simulink model "Tisch"  (R2016b)
settings: Solver=VariableStepAuto  StartTime=0.0  StopTime=5  RelTol=1e-3
settings Model: Creator=fabienlapok  LastModifiedBy=fabienlapok

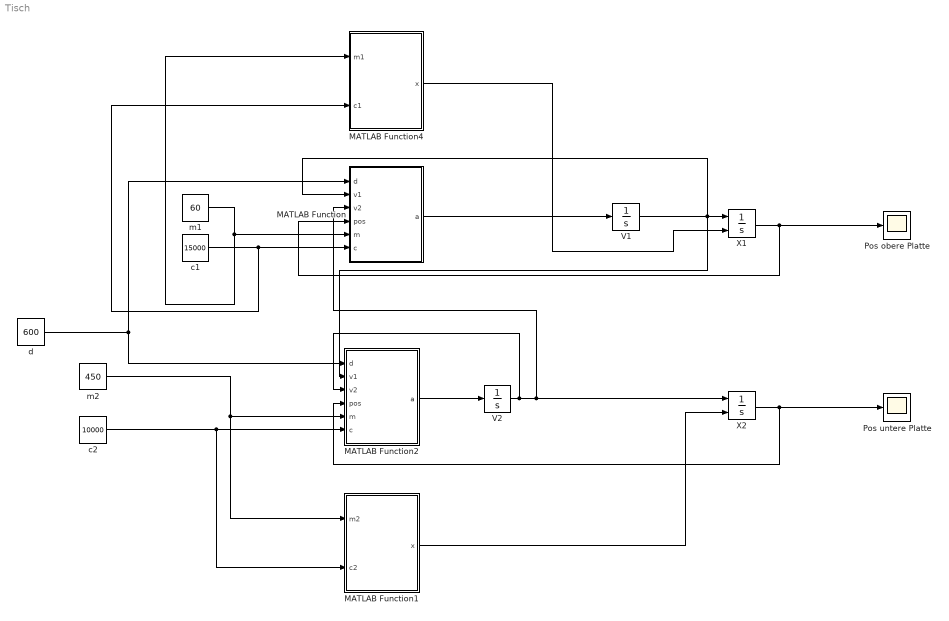
== system Tisch ==
  MATLAB Function : MATLAB Function  TreatAsAtomicUnit=on
  MATLAB Function1 : MATLAB Function  TreatAsAtomicUnit=on
  MATLAB Function2 : MATLAB Function  TreatAsAtomicUnit=on
  MATLAB Function4 : MATLAB Function  TreatAsAtomicUnit=on
  Pos obere Platte : Scope
  Pos untere Platte : Scope
  V1 : Integrator
  V2 : Integrator
  X1 : Integrator  InitialConditionSource=external
  X2 : Integrator  InitialConditionSource=external
  c1 : Constant  Value=15000
  c2 : Constant  Value=10000
  d : Constant  Value=600
  m1 : Constant  Value=60
  m2 : Constant  Value=450
  wires:
  MATLAB Function2/1(a) -> V2/1
  V2/1 -> MATLAB Function2/3(v2), MATLAB Function/3(v2), X2/1
  MATLAB Function/1(a) -> V1/1
  d/1 -> MATLAB Function/1(d), MATLAB Function2/1(d)
  m1/1 -> MATLAB Function4/1(m1), MATLAB Function/5(m)
  m2/1 -> MATLAB Function1/1(m2), MATLAB Function2/5(m)
  c1/1 -> MATLAB Function4/2(c1), MATLAB Function/6(c)
  c2/1 -> MATLAB Function1/2(c2), MATLAB Function2/6(c)
  X2/1 -> Pos untere Platte/1, MATLAB Function2/4(pos)
  X1/1 -> MATLAB Function/4(pos), Pos obere Platte/1
  MATLAB Function4/1(x) -> X1/2
  MATLAB Function1/1(x) -> X2/2
  V1/1 -> MATLAB Function2/2(v1), X1/1, MATLAB Function/2(v1)

== matlab function Tisch/MATLAB Function1 ==
  data: x output; m2 input; c2 input
function x = RuheposM2(m2, c2)
%Funktion zur Berechnung der Ruheposition der ersten (oberen) Platte 
    g= -9.81;
    
    x = m2*g/(2*c2); %[m]

== matlab function Tisch/MATLAB Function ==
  data: d input; a output; v1 input; v2 input; pos input; m input; c input
function a = BeschlM1(d, v1,v2, pos, m, c)
%Funktion zur Berechnung der Beschleunigung der oberen Platte 
    
    g= -9.81; %[m/s^2]
    
    % Dämpfkraft die auf die Platte in Abhängigkeit der Bewegung wirkt 
    Fd = -d * (v1-v2); %[kg*m/s^2]
    
    % Federkraft, die auf die Platte wirkt
    Ff = -c * (pos - 0.001); %[kg*m/s^2]
    
    % Gewichtskraft die auf die Platte wirkt
    Fg = m * g; %[kg*m/s]
    
    % Beschläunigung 
    a = (2 * (Ff+Fd) + Fg) / m; %[m/s]

== matlab function Tisch/MATLAB Function2 ==
  data: d input; a output; v1 input; v2 input; pos input; m input; c input
function a = BeschlM2(d, v1,v2, pos, m, c)
%Funktion zur Berechnung der Beschleunigung der unteren Platte 
    g= -9.81; %[m/s^2]
    
    % Dämpfkraft die auf die Platte in Abhängigkeit der Bewegung wirkt 
    Fd = -d * (v2-v1); %[kg*m/s^2]
    
    % Federkraft, die auf die Platte wirkt
    Ff = -c * (pos - 0.001); %[kg*m/s^2]
    
    % Gewichtskraft die auf die Platte wirkt
    Fg = m*g; %[kg*m/s]
    
    % Beschläunigung 
    a = (2 * (Ff+Fd) + Fg) / m; %[m/s]

== matlab function Tisch/MATLAB Function4 ==
  data: x output; m1 input; c1 input
function x = RuheposM1(m1, c1)
%Funktion zur Berechnung der Ruheposition der ersten (oberen) Platte 
    g= -9.81;
    
    x = m1 * g / (2*c1); %[m]
